simulink model "Model1"  (R2018b)
settings: Solver=ode8  StartTime=0.0  StopTime=100.0  FixedStep=0.01  RelTol=1e-6
settings Model: SimulationMode=accelerator  Creator=claudio.menghi  LastModifiedBy=claudio.menghi
settings SolverCC: MaxConsecutiveZCs=10000  ShapePreserveControl=EnableAll  ZeroCrossControl=EnableAll  ZeroCrossAlgorithm=Adaptive  AutoInsertRateTranBlk=on

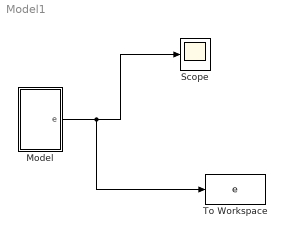
== system Model1 ==
  Model : Subsystem
  Scope : Scope
  To Workspace : ToWorkspace  VariableName=e  SaveFormat=Timeseries  SampleTime=-1
  wires:
  Model/1(e) -> To Workspace/1, Scope/1

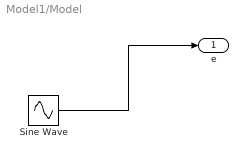
== system Model1/Model ==
  Sine Wave : Sin  Amplitude=2  SampleTime=0
  e : Outport
  wires:
  Sine Wave/1 -> e/1
